simulink model "ex4_4_3"  (Simulink 7.4)
settings: Solver=ode4  StartTime=0.0  StopTime=1  FixedStep=0.01  RelTol=1e-3
values from neighbouring files (symbols this model uses):
  A = [ 0 1; -2 -3 ]    [ex4_4_1_1.m]    (also in ex4_4_1_2.m = [ 0 1 1; -2 -3 1; 1 0 0]; ex4_4_2.m = [ -3 1; 2 -2 ])
  B = [ 1; 0 ]    [ex4_4_1_1.m]    (also in ex4_4_1_2.m = [ 0 1; 1 0; 0 0 ]; ex4_4_2.m = [ 2; 0 ])
  K = subs([k1 k2], {p1, p2}, {-8+4j,-8-4j})    [ex4_4_2.m]
undefined symbols (not defined in the file or in its folder): x0
settings Model: Creator=student  LastModifiedBy=student

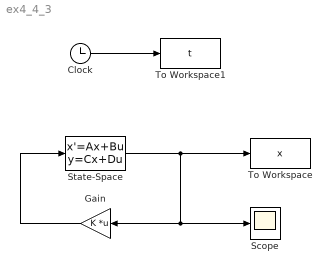
== system ex4_4_3 ==
  Clock : Clock
      settings: Decimation=10
  Gain : Gain  Gain=K  Multiplication=Matrix(K*u)  ParameterDataType=fixdt(1, 16)  ParameterScaling=2^0  OutDataType=fixdt(1, 16)  OutScaling=2^0
  Scope : Scope
  State-Space : StateSpace  A=A  B=B  C=eye(2)  D=zeros(2,1)  X0=x0
  To Workspace : ToWorkspace  VariableName=x  SampleTime=-1  SaveFormat=Array
  To Workspace1 : ToWorkspace  VariableName=t  SampleTime=-1  SaveFormat=Array
  wires:
  State-Space/1 -> To Workspace/1, Scope/1, Gain/1
  Gain/1 -> State-Space/1
  Clock/1 -> To Workspace1/1
